simulink model "Jenny3"  (R2013b)
settings: Solver=ode45  StartTime=0.0  StopTime=inf  RelTol=1e-3
undefined symbols (not defined in the file): CR, LF, serial
libraries: instrumentlib x2, simulink x1
settings Model: Creator=frf  LastModifiedBy=user
settings DataIOCC: MaxDataPoints=10000  SignalLoggingSaveFormat=ModelDataLogs
settings DebuggingCC: MultiTaskDSMMsg=warning  MultiTaskCondExecSysMsg=none  StateNameClashWarn=warning
settings HardwareCC: ProdLargestAtomicFloat=Double
settings RTWCC: IncludeERTFirstTime=on

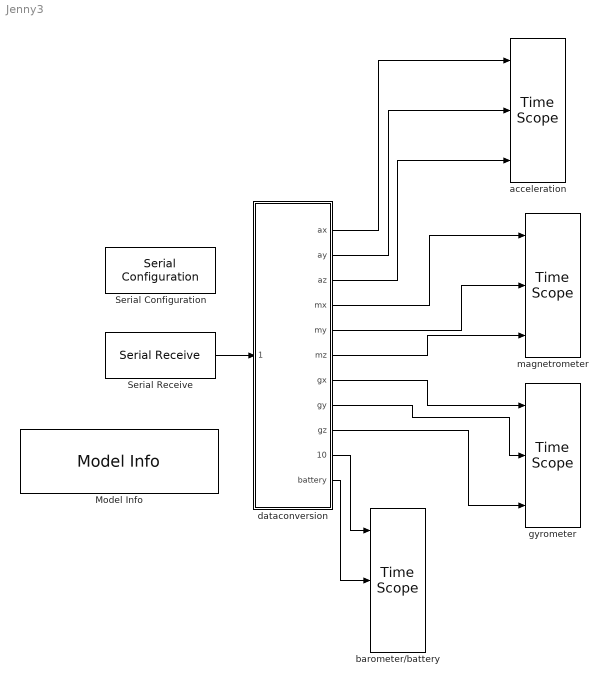
== system Jenny3 ==
  Model Info : simulink/Model-Wide Utilities/Model Info  InitialBlockCM=None  BlockCM=None  Frame=on  DisplayStringWithTags=|  HorizontalTextAlignment=Left  LeftAlignmentValue=0.02  SourceBlockDiagram=kalibrering_6deg  TagMaxNumber=20
      | The sample time must also be defined. 
      | Both in serial recieve and A block
      | 
      | Name: Ts
  Serial Configuration : instrumentlib/Serial Configuration  Priority=-200000  ComPortMenu=COM16  ComPort=COM16  ObjConstructor=serial('COM16');  BaudRate=9600  DataBits=8  Parity=none  StopBits=1  FlowControl=none  Timeout=1000000  ByteOrder=LittleEndian
  Serial Receive : instrumentlib/Serial Receive  ComPortMenu=COM16  ComPort=COM16  ObjConstructor=serial('COM16');  Terminator=CR/LF ('\r\n')  DataSize="[12   1]"  DataType=int32  EnableBlockingMode=on  ActionDataUnavailable=Error  CustomValue=0  SampleTime=1000
  acceleration : TimeScope  NumInputPorts=3  DefaultConfigurationName=spbscopes.TimeScopeBlockCfg
      settings: CopyFcn=scopeextensions.ScopeBlock.onCoreBlockCopy(gcbh);  DeleteFcn=scopeextensions.ScopeBlock.callback(gcbh, 'onBlockDelete');  PreSaveFcn=scopeextensions.ScopeBlock.callback(gcbh, 'onModelSave');  NameChangeFcn=scopeextensions.ScopeBlock.callback(gcbh, 'onBlockRename');  DestroyFcn=scopeextensions.ScopeBlock.onBlockDestroy(gcbh)  CloseFcn=scopeextensions.ScopeBlock.callback(gcbh, 'onBlockClose');  PreDeleteFcn=scopeextensions.ScopeBlock.callback(gcbh, 'onBlockPreDelete');
  barometer/battery : TimeScope  NumInputPorts=3  DefaultConfigurationName=spbscopes.TimeScopeBlockCfg
      settings: CopyFcn=scopeextensions.ScopeBlock.onCoreBlockCopy(gcbh);  DeleteFcn=scopeextensions.ScopeBlock.callback(gcbh, 'onBlockDelete');  PreSaveFcn=scopeextensions.ScopeBlock.callback(gcbh, 'onModelSave');  NameChangeFcn=scopeextensions.ScopeBlock.callback(gcbh, 'onBlockRename');  DestroyFcn=scopeextensions.ScopeBlock.onBlockDestroy(gcbh)  CloseFcn=scopeextensions.ScopeBlock.callback(gcbh, 'onBlockClose');  PreDeleteFcn=scopeextensions.ScopeBlock.callback(gcbh, 'onBlockPreDelete');
  dataconversion : Subsystem
  gyrometer : TimeScope  NumInputPorts=3  DefaultConfigurationName=spbscopes.TimeScopeBlockCfg
      settings: CopyFcn=scopeextensions.ScopeBlock.onCoreBlockCopy(gcbh);  DeleteFcn=scopeextensions.ScopeBlock.callback(gcbh, 'onBlockDelete');  PreSaveFcn=scopeextensions.ScopeBlock.callback(gcbh, 'onModelSave');  NameChangeFcn=scopeextensions.ScopeBlock.callback(gcbh, 'onBlockRename');  DestroyFcn=scopeextensions.ScopeBlock.onBlockDestroy(gcbh)  CloseFcn=scopeextensions.ScopeBlock.callback(gcbh, 'onBlockClose');  PreDeleteFcn=scopeextensions.ScopeBlock.callback(gcbh, 'onBlockPreDelete');
  magnetrometer : TimeScope  NumInputPorts=3  DefaultConfigurationName=spbscopes.TimeScopeBlockCfg
      settings: CopyFcn=scopeextensions.ScopeBlock.onCoreBlockCopy(gcbh);  DeleteFcn=scopeextensions.ScopeBlock.callback(gcbh, 'onBlockDelete');  PreSaveFcn=scopeextensions.ScopeBlock.callback(gcbh, 'onModelSave');  NameChangeFcn=scopeextensions.ScopeBlock.callback(gcbh, 'onBlockRename');  DestroyFcn=scopeextensions.ScopeBlock.onBlockDestroy(gcbh)  CloseFcn=scopeextensions.ScopeBlock.callback(gcbh, 'onBlockClose');  PreDeleteFcn=scopeextensions.ScopeBlock.callback(gcbh, 'onBlockPreDelete');
  wires:
  Serial Receive/1 -> dataconversion/1(11 x uint8)
  dataconversion/1(ax) -> acceleration/1
  dataconversion/2(ay) -> acceleration/2
  dataconversion/3(az) -> acceleration/3
  dataconversion/4(mx) -> magnetrometer/1
  dataconversion/5(my) -> magnetrometer/2
  dataconversion/6(mz) -> magnetrometer/3
  dataconversion/7(gx) -> gyrometer/1
  dataconversion/8(gy) -> gyrometer/2
  dataconversion/9(gz) -> gyrometer/3
  dataconversion/10(barometer) -> barometer/battery/1
  dataconversion/11(battery) -> barometer/battery/2

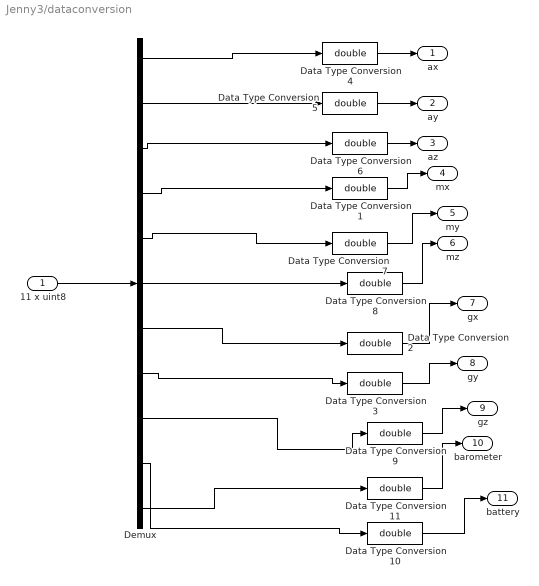
== system Jenny3/dataconversion ==
  11 x uint8 : Inport
  Data Type Conversion{1..11} (11 alike) : DataTypeConversion  OutDataTypeStr=double  SaturateOnIntegerOverflow=on  RndMeth=Zero
  Demux : Demux  Outputs=11
  ax : Outport
  ay : Outport  Port=2
  az : Outport  Port=3
  mx : Outport  Port=4
  my : Outport  Port=5
  mz : Outport  Port=6
  gx : Outport  Port=7
  gy : Outport  Port=8
  gz : Outport  Port=9
  barometer : Outport  Port=10
  battery : Outport  Port=11
  wires:
  11 x uint8/1 -> Demux/1
  Demux/1 -> Data Type Conversion4/1
  Demux/2 -> Data Type Conversion5/1
  Demux/3 -> Data Type Conversion6/1
  Data Type Conversion6/1 -> az/1
  Data Type Conversion5/1 -> ay/1
  Data Type Conversion4/1 -> ax/1
  Demux/5 -> Data Type Conversion7/1
  Demux/6 -> Data Type Conversion8/1
  Data Type Conversion8/1 -> mz/1
  Data Type Conversion7/1 -> my/1
  Demux/4 -> Data Type Conversion1/1
  Data Type Conversion1/1 -> mx/1
  Demux/8 -> Data Type Conversion3/1
  Demux/7 -> Data Type Conversion2/1
  Demux/10 -> Data Type Conversion10/1
  Demux/9 -> Data Type Conversion9/1
  Demux/11 -> Data Type Conversion11/1
  Data Type Conversion2/1 -> gx/1
  Data Type Conversion3/1 -> gy/1
  Data Type Conversion9/1 -> gz/1
  Data Type Conversion11/1 -> barometer/1
  Data Type Conversion10/1 -> battery/1
